simulink model "relative_gain_array_example_lti_system"  (R2024a)
settings: Solver=VariableStepAuto  StartTime=0.0  StopTime=80  RelTol=1e-3
libraries: cstblocks x1
settings Model: Creator=Ranjeet  LastModifiedBy=Ranjeet
settings DataIOCC: SaveOutput=off  SaveTime=off  ReturnWorkspaceOutputs=off

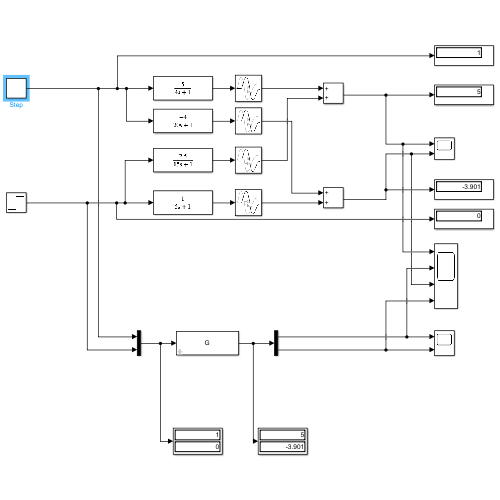
[thumbnail: Simulink's stored preview of the top-level diagram]
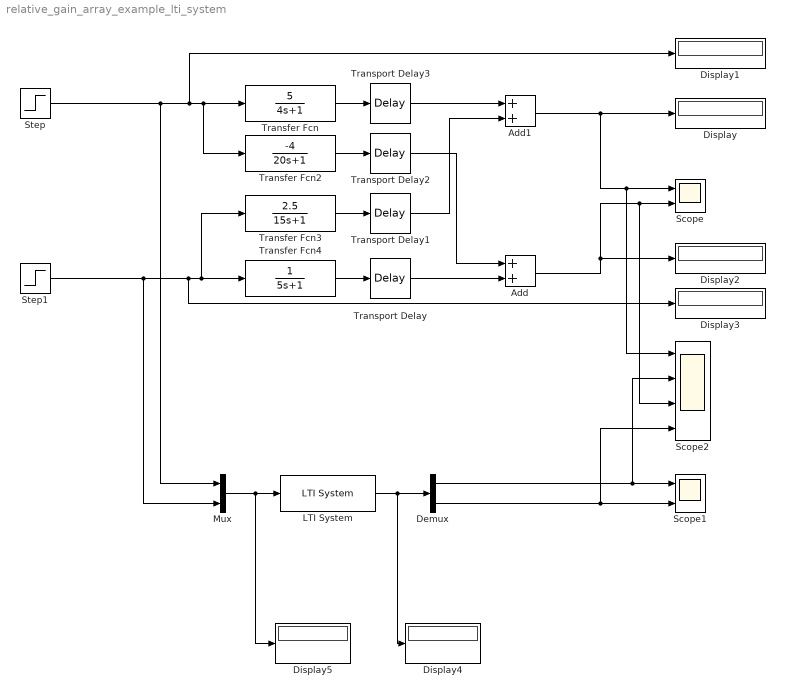
== system relative_gain_array_example_lti_system ==
  Add : Sum
  Add1 : Sum
  Demux : Demux  Outputs=2
  Display{,1..5} (6 alike) : Display
  LTI System : cstblocks/LTI System  sys=G  IC=[]  PadeOrder=1
  Mux : Mux  Inputs=2
  Scope : Scope  NumInputPorts=2
  Scope1 : Scope  NumInputPorts=2
  Scope2 : Scope  NumInputPorts=4
  Step : Step  Time=0  SampleTime=0
  Step1 : Step  Time=0  After=0  SampleTime=0
  Transfer Fcn : TransferFcn  Numerator=[5]  Denominator=[4 1]
  Transfer Fcn2 : TransferFcn  Numerator=[-4]  Denominator=[20 1]
  Transfer Fcn3 : TransferFcn  Numerator=[2.5]  Denominator=[15 1]
  Transfer Fcn4 : TransferFcn  Denominator=[5 1]
  Transport Delay : TransportDelay
  Transport Delay1 : TransportDelay  DelayTime=5
  Transport Delay2 : TransportDelay  DelayTime=6
  Transport Delay3 : TransportDelay  DelayTime=3
  wires:
  Step/1 -> Mux/1, Display1/1, Transfer Fcn2/1, Transfer Fcn/1
  Step1/1 -> Mux/2, Display3/1, Transfer Fcn3/1, Transfer Fcn4/1
  Transfer Fcn4/1 -> Transport Delay/1
  Transfer Fcn/1 -> Transport Delay3/1
  Transfer Fcn2/1 -> Transport Delay2/1
  Transfer Fcn3/1 -> Transport Delay1/1
  Add1/1 -> Scope2/1, Scope/1, Display/1
  Add/1 -> Display2/1, Scope2/3, Scope/2
  Mux/1 -> Display5/1, LTI System/1
  LTI System/1 -> Display4/1, Demux/1
  Demux/1 -> Scope2/2, Scope1/1
  Demux/2 -> Scope2/4, Scope1/2
  Transport Delay/1 -> Add/2
  Transport Delay1/1 -> Add1/2
  Transport Delay2/1 -> Add/1
  Transport Delay3/1 -> Add1/1
